simulink model "baseModel"  (R2018a)
settings: Solver=VariableStepAuto  StartTime=0.0  StopTime=300  RelTol=1e-3
values from neighbouring files (symbols this model uses):
  des_distance = 5    [Load_Parameters.m]
  init_speed = 10    [Load_Parameters.m]
  K_LQR = [0.447 1.689 0.625]    [Load_Parameters.m]
  vehicle_T = 0.4    [Load_Parameters.m]
settings Model: Creator=Manchey  LastModifiedBy=Manchey

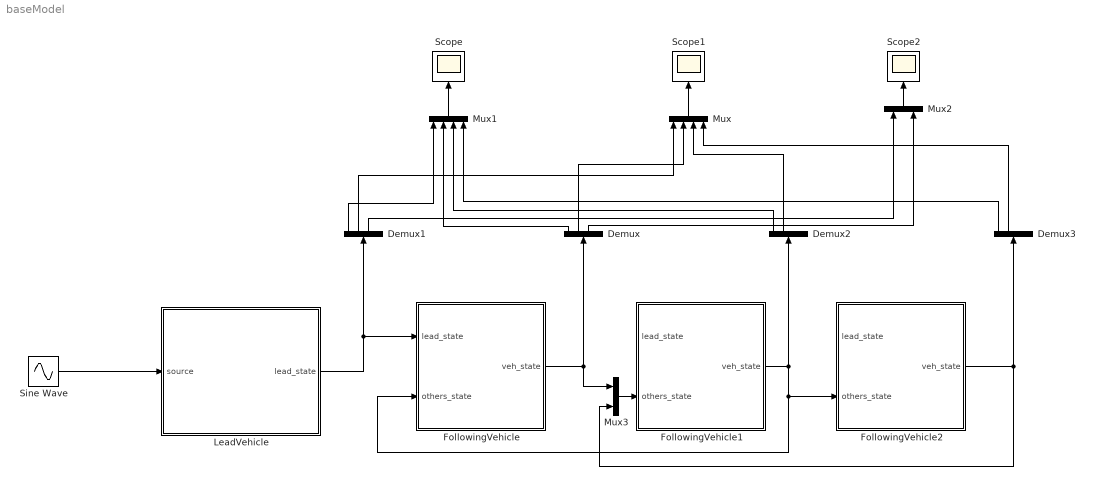
== system baseModel ==
  Demux{,1..3} (4 alike) : Demux
  FollowingVehicle : Subsystem
  FollowingVehicle1 : Subsystem
  FollowingVehicle2 : Subsystem
  LeadVehicle : Subsystem
  Mux : Mux
  Mux1 : Mux
  Mux2 : Mux  Inputs=2
  Mux3 : Mux  Inputs=2
  Scope : Scope
  Scope1 : Scope
  Scope2 : Scope
  Sine Wave : Sin  Amplitude=2  Bias=10  Frequency=0.05  SampleTime=0
  wires:
  LeadVehicle/1(lead_state) -> FollowingVehicle/1(lead_state), Demux1/1
  FollowingVehicle/1(veh_state) -> Mux3/1, Demux/1
  Demux1/2 -> Mux/1
  Demux/2 -> Mux/2
  Demux1/1 -> Mux1/1
  Demux/1 -> Mux1/2
  FollowingVehicle1/1(veh_state) -> FollowingVehicle/2(others_state), FollowingVehicle2/2(others_state), Demux2/1
  FollowingVehicle2/1(veh_state) -> Mux3/2, Demux3/1
  Demux2/2 -> Mux/3
  Demux3/2 -> Mux/4
  Demux2/1 -> Mux1/3
  Demux3/1 -> Mux1/4
  Mux1/1 -> Scope/1
  Mux/1 -> Scope1/1
  Mux2/1 -> Scope2/1
  Demux1/3 -> Mux2/1
  Demux/3 -> Mux2/2
  Sine Wave/1 -> LeadVehicle/1(source)
  Mux3/1 -> FollowingVehicle1/2(others_state)

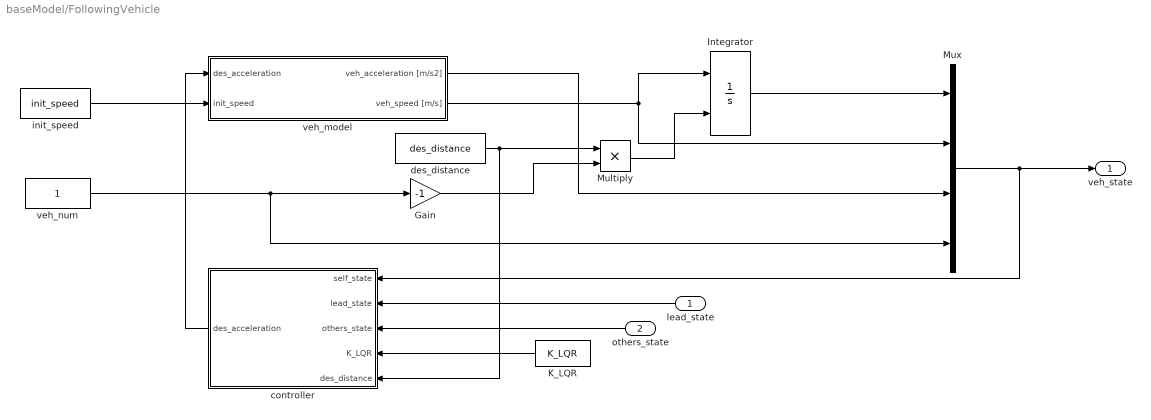
== system baseModel/FollowingVehicle ==
  lead_state : Inport
  others_state : Inport  Port=2
  Gain : Gain  Gain=-1
  Integrator : Integrator  InitialConditionSource=external
  K_LQR : Constant  Value=K_LQR
  Multiply : Product
  Mux : Mux
  controller : MATLAB Function  TreatAsAtomicUnit=on
  des_distance : Constant  Value=des_distance
  init_speed : Constant  Value=init_speed
  veh_model : Subsystem
  veh_num : Constant
  veh_state : Outport
  wires:
  controller/1(des_acceleration) -> veh_model/1(des_acceleration)
  veh_model/1(veh_acceleration [m/s2]) -> Mux/3
  Mux/1 -> veh_state/1, controller/1(self_state)
  Integrator/1 -> Mux/1
  init_speed/1 -> veh_model/2(init_speed)
  veh_num/1 -> Gain/1, Mux/4
  veh_model/2(veh_speed [m/s]) -> Integrator/1, Mux/2
  Multiply/1 -> Integrator/2
  des_distance/1 -> controller/5(des_distance), Multiply/1
  Gain/1 -> Multiply/2
  lead_state/1 -> controller/2(lead_state)
  others_state/1 -> controller/3(others_state)
  K_LQR/1 -> controller/4(K_LQR)

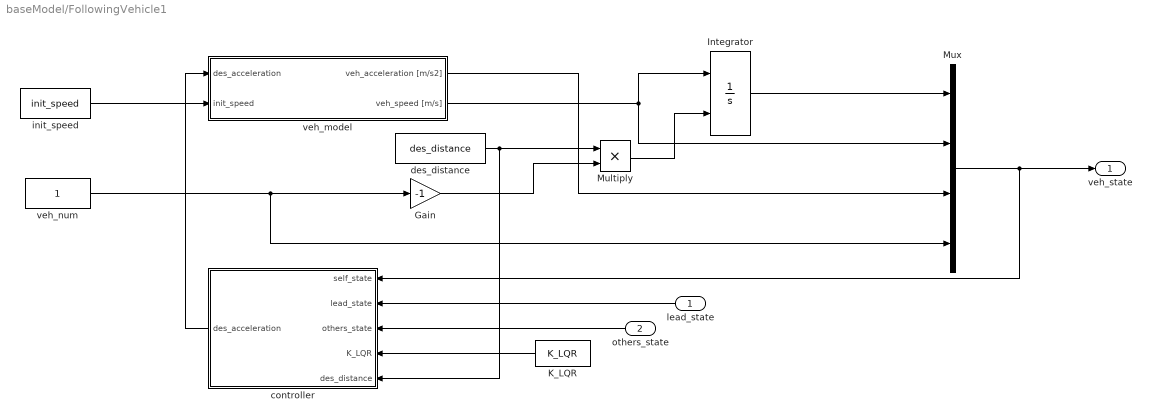
== system baseModel/FollowingVehicle1 ==
  lead_state : Inport
  others_state : Inport  Port=2
  Gain : Gain  Gain=-1
  Integrator : Integrator  InitialConditionSource=external
  K_LQR : Constant  Value=K_LQR
  Multiply : Product
  Mux : Mux
  controller : MATLAB Function  TreatAsAtomicUnit=on
  des_distance : Constant  Value=des_distance
  init_speed : Constant  Value=init_speed
  veh_model : Subsystem
  veh_num : Constant
  veh_state : Outport
  wires:
  controller/1(des_acceleration) -> veh_model/1(des_acceleration)
  veh_model/1(veh_acceleration [m/s2]) -> Mux/3
  Mux/1 -> veh_state/1, controller/1(self_state)
  Integrator/1 -> Mux/1
  init_speed/1 -> veh_model/2(init_speed)
  veh_num/1 -> Gain/1, Mux/4
  veh_model/2(veh_speed [m/s]) -> Integrator/1, Mux/2
  Multiply/1 -> Integrator/2
  des_distance/1 -> controller/5(des_distance), Multiply/1
  Gain/1 -> Multiply/2
  lead_state/1 -> controller/2(lead_state)
  others_state/1 -> controller/3(others_state)
  K_LQR/1 -> controller/4(K_LQR)

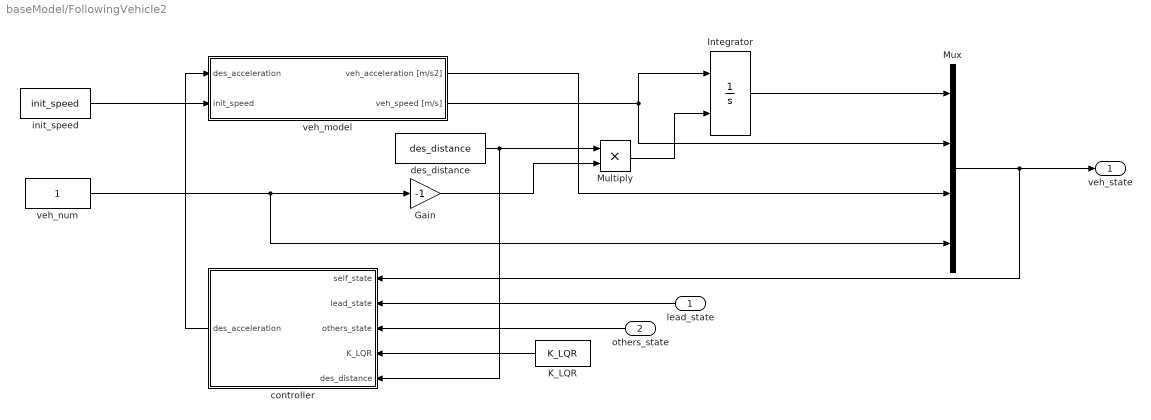
== system baseModel/FollowingVehicle2 ==
  lead_state : Inport
  others_state : Inport  Port=2
  Gain : Gain  Gain=-1
  Integrator : Integrator  InitialConditionSource=external
  K_LQR : Constant  Value=K_LQR
  Multiply : Product
  Mux : Mux
  controller : MATLAB Function  TreatAsAtomicUnit=on
  des_distance : Constant  Value=des_distance
  init_speed : Constant  Value=init_speed
  veh_model : Subsystem
  veh_num : Constant
  veh_state : Outport
  wires:
  controller/1(des_acceleration) -> veh_model/1(des_acceleration)
  veh_model/1(veh_acceleration [m/s2]) -> Mux/3
  Mux/1 -> veh_state/1, controller/1(self_state)
  Integrator/1 -> Mux/1
  init_speed/1 -> veh_model/2(init_speed)
  veh_num/1 -> Gain/1, Mux/4
  veh_model/2(veh_speed [m/s]) -> Integrator/1, Mux/2
  Multiply/1 -> Integrator/2
  des_distance/1 -> controller/5(des_distance), Multiply/1
  Gain/1 -> Multiply/2
  lead_state/1 -> controller/2(lead_state)
  others_state/1 -> controller/3(others_state)
  K_LQR/1 -> controller/4(K_LQR)

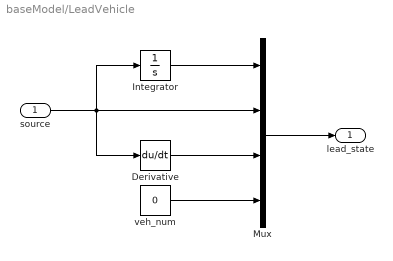
== system baseModel/LeadVehicle ==
  source : Inport
  Derivative : Derivative
  Integrator : Integrator
  Mux : Mux
  veh_num : Constant  Value=0
  lead_state : Outport
  wires:
  Mux/1 -> lead_state/1
  Integrator/1 -> Mux/1
  source/1 -> Derivative/1, Mux/2, Integrator/1
  Derivative/1 -> Mux/3
  veh_num/1 -> Mux/4

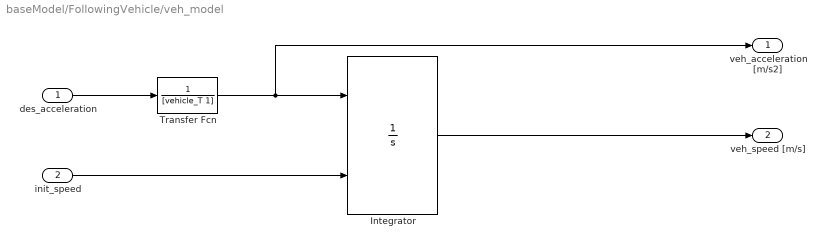
== system baseModel/FollowingVehicle/veh_model ==
  des_acceleration : Inport
  init_speed : Inport  Port=2
  Integrator : Integrator  InitialConditionSource=external  LimitOutput=on  UpperSaturationLimit=100  LowerSaturationLimit=0
  Transfer Fcn : TransferFcn  Denominator=[vehicle_T 1]
  veh_acceleration [m/s2] : Outport
  veh_speed [m/s] : Outport  Port=2
  wires:
  des_acceleration/1 -> Transfer Fcn/1
  Transfer Fcn/1 -> veh_acceleration [m/s2]/1, Integrator/1
  init_speed/1 -> Integrator/2
  Integrator/1 -> veh_speed [m/s]/1

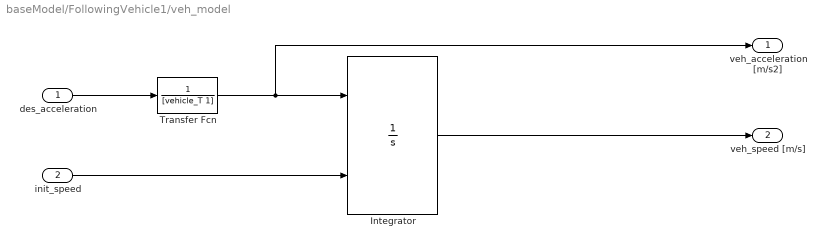
== system baseModel/FollowingVehicle1/veh_model ==
  des_acceleration : Inport
  init_speed : Inport  Port=2
  Integrator : Integrator  InitialConditionSource=external  LimitOutput=on  UpperSaturationLimit=100  LowerSaturationLimit=0
  Transfer Fcn : TransferFcn  Denominator=[vehicle_T 1]
  veh_acceleration [m/s2] : Outport
  veh_speed [m/s] : Outport  Port=2
  wires:
  des_acceleration/1 -> Transfer Fcn/1
  Transfer Fcn/1 -> veh_acceleration [m/s2]/1, Integrator/1
  init_speed/1 -> Integrator/2
  Integrator/1 -> veh_speed [m/s]/1

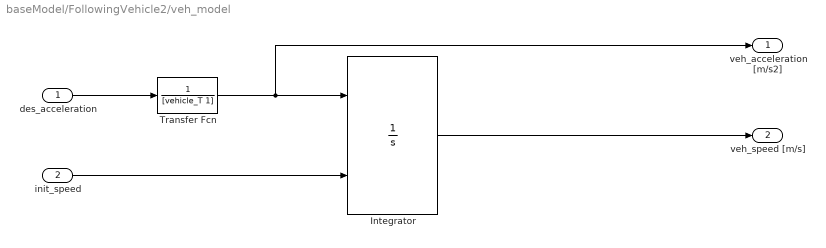
== system baseModel/FollowingVehicle2/veh_model ==
  des_acceleration : Inport
  init_speed : Inport  Port=2
  Integrator : Integrator  InitialConditionSource=external  LimitOutput=on  UpperSaturationLimit=100  LowerSaturationLimit=0
  Transfer Fcn : TransferFcn  Denominator=[vehicle_T 1]
  veh_acceleration [m/s2] : Outport
  veh_speed [m/s] : Outport  Port=2
  wires:
  des_acceleration/1 -> Transfer Fcn/1
  Transfer Fcn/1 -> veh_acceleration [m/s2]/1, Integrator/1
  init_speed/1 -> Integrator/2
  Integrator/1 -> veh_speed [m/s]/1

== matlab function baseModel/FollowingVehicle/controller ==
  data: self_state input; des_acceleration output; lead_state input; others_state input; K_LQR input; des_distance input
function des_acceleration = fcn(self_state, lead_state, others_state, K_LQR, des_distance)
%%%Function:
%   Calculate desired acceleration

%%%Arguments:
%   self_state = [self_position; self_speed; self_acceleration; self_num]
%   lead_state = [lead_position; lead_speed; lead_acceleration; 0]
%   others_state = [other_x; other_v; other_a; %other_num; ... ]
%   K_LQR = [k1 k2 k3]

%%%Outputs:
%   desired acceleration


%% Initial Parameters
K_LQR_ = [K_LQR' K_LQR(1)*des_distance]; 

%% Control Input from Lead Vehicle
if length(lead_state) == 1
    ctrl_lead = 0;
else
    ctrl_lead = K_LQR_ * (lead_state - self_state);
end

%% Control Input from V2V
num_others = length(others_state)/4;
ctrl_others=0;
if num_others >= 1
    for i = 1:num_others
        ctrl_others = ctrl_others + K_LQR_ * (others_state(1+(i-1)*4:4+(i-1)*4)-self_state);
    end
end

%% Sum of control signals
des_acceleration = ctrl_lead + ctrl_others;

== matlab function baseModel/FollowingVehicle1/controller ==
  data: self_state input; des_acceleration output; lead_state input; others_state input; K_LQR input; des_distance input
function des_acceleration = fcn(self_state, lead_state, others_state, K_LQR, des_distance)
%%%Function:
%   Calculate desired acceleration

%%%Arguments:
%   self_state = [self_position; self_speed; self_acceleration; self_num]
%   lead_state = [lead_position; lead_speed; lead_acceleration; 0]
%   others_state = [other_x; other_v; other_a; %other_num; ... ]
%   K_LQR = [k1 k2 k3]

%%%Outputs:
%   desired acceleration


%% Initial Parameters
K_LQR_ = [K_LQR' K_LQR(1)*des_distance]; 

%% Control Input from Lead Vehicle
if length(lead_state) == 1
    ctrl_lead = 0;
else
    ctrl_lead = K_LQR_ * (lead_state - self_state);
end

%% Control Input from V2V
num_others = length(others_state)/4;
ctrl_others=0;
if num_others >= 1
    for i = 1:num_others
        ctrl_others = ctrl_others + K_LQR_ * (others_state(1+(i-1)*4:4+(i-1)*4)-self_state);
    end
end

%% Sum of control signals
des_acceleration = ctrl_lead + ctrl_others;

== matlab function baseModel/FollowingVehicle2/controller ==
  data: self_state input; des_acceleration output; lead_state input; others_state input; K_LQR input; des_distance input
function des_acceleration = fcn(self_state, lead_state, others_state, K_LQR, des_distance)
%%%Function:
%   Calculate desired acceleration

%%%Arguments:
%   self_state = [self_position; self_speed; self_acceleration; self_num]
%   lead_state = [lead_position; lead_speed; lead_acceleration; 0]
%   others_state = [other_x; other_v; other_a; %other_num; ... ]
%   K_LQR = [k1 k2 k3]

%%%Outputs:
%   desired acceleration


%% Initial Parameters
K_LQR_ = [K_LQR' K_LQR(1)*des_distance]; 

%% Control Input from Lead Vehicle
if length(lead_state) == 1
    ctrl_lead = 0;
else
    ctrl_lead = K_LQR_ * (lead_state - self_state);
end

%% Control Input from V2V
num_others = length(others_state)/4;
ctrl_others=0;
if num_others >= 1
    for i = 1:num_others
        ctrl_others = ctrl_others + K_LQR_ * (others_state(1+(i-1)*4:4+(i-1)*4)-self_state);
    end
end

%% Sum of control signals
des_acceleration = ctrl_lead + ctrl_others;
